simulink model "system_level_0317"  (R2025a)
settings: Solver=VariableStepAuto  StartTime=0.0  StopTime=600  RelTol=1e-3
libraries: simulink x6
settings Model: PacingRate=40  Creator=lynnyu  LastModifiedBy=lynnyu

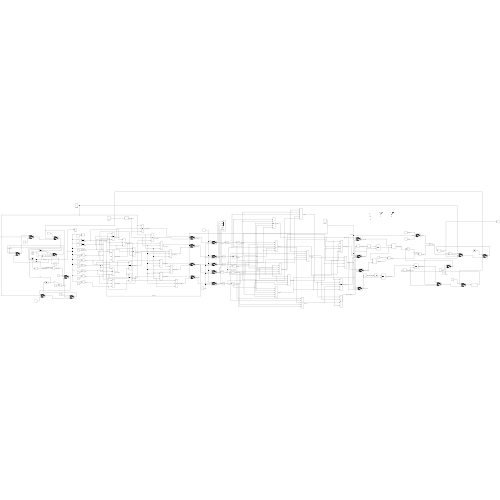
[thumbnail: Simulink's stored preview of the top-level diagram]
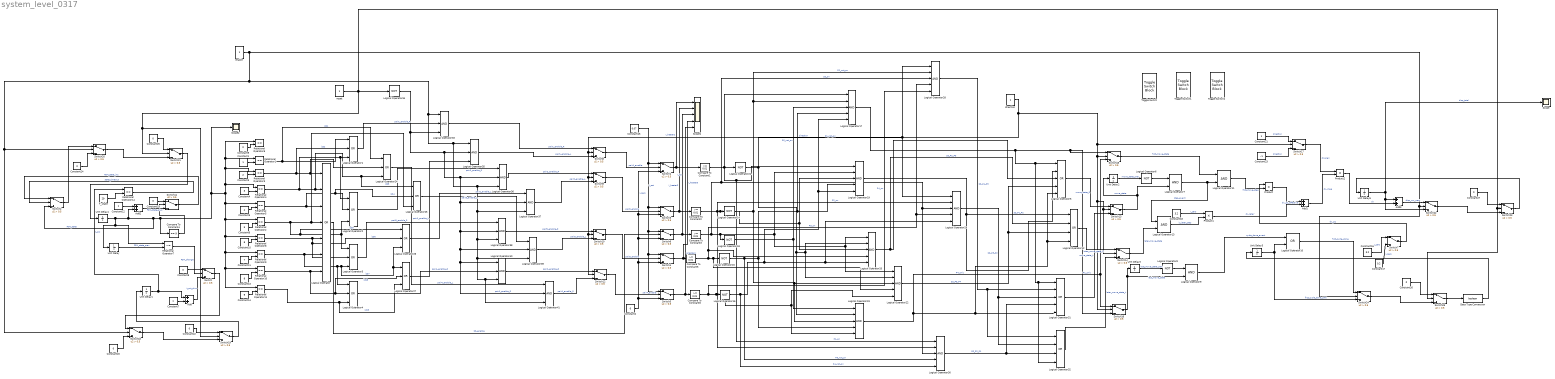
== system system_level_0317 ==
  Add{,1..3} (4 alike) : Sum
  Compare To Constant{1..3,5..6} (5 alike) : simulink/Logic and Bit Operations/Compare To Constant  relop=>=  const=0.01  OutDataTypeStr=boolean
  Compare To Constant4 : simulink/Logic and Bit Operations/Compare To Constant  relop===  const=9  OutDataTypeStr=boolean
  Constant{1,7,12,21} (4 alike) : Constant
  Constant10 : Constant  Value=6
  Constant11 : Constant  Value=7
  Constant13 : Constant  Value=8
  Constant14 : Constant  Value=9
  Constant15 : Constant  Value=0.07
  Constant16 : Constant  Value=3.2
  Constant17 : Constant  Value=0.2
  Constant18 : Constant  Value=3.2
  Constant{2,8..9,19..20,22,24..27} (10 alike) : Constant  Value=0
  Constant23 : Constant  Value=-1
  Constant3 : Constant  Value=2
  Constant4 : Constant  Value=3
  Constant5 : Constant  Value=4
  Constant6 : Constant  Value=5
  Data Type Conversion : DataTypeConversion  OutDataTypeStr=boolean  SaturateOnIntegerOverflow=off  RndMeth=Floor
  Logical Operator : Logic  Operator=OR  Inputs=7  AllPortsSameDT=off  OutDataTypeStr=boolean
  Logical Operator{1..4,24..27} (8 alike) : Logic  Operator=OR  Inputs=3  AllPortsSameDT=off  OutDataTypeStr=boolean
  Logical Operator10 : Logic  Operator=OR  AllPortsSameDT=off  OutDataTypeStr=boolean
  Logical Operator{7,9,11,13} (4 alike) : Logic  AllPortsSameDT=off  OutDataTypeStr=boolean
  Logical Operator12 : Logic  Operator=OR  Inputs=4  AllPortsSameDT=off  OutDataTypeStr=boolean
  Logical Operator{14..16,18,21,34} (6 alike) : Logic  Operator=NOT  Inputs=3  AllPortsSameDT=off  OutDataTypeStr=boolean
  Logical Operator{17,19..20,22..23,28..30} (8 alike) : Logic  Inputs=5  AllPortsSameDT=off  OutDataTypeStr=boolean
  Logical Operator31 : Logic  Operator=OR  Inputs=5  AllPortsSameDT=off  OutDataTypeStr=boolean
  Logical Operator32 : Logic  Operator=OR  Inputs=4  AllPortsSameDT=off  OutDataTypeStr=boolean
  Logical Operator{33,35..41} (8 alike) : Logic  Inputs=3  AllPortsSameDT=off  OutDataTypeStr=boolean
  Logical Operator5 : Logic  Operator=OR  Inputs=5  AllPortsSameDT=off  OutDataTypeStr=boolean
  Logical Operator6 : Logic  Operator=NOT  Inputs=5  AllPortsSameDT=off  OutDataTypeStr=boolean
  Logical Operator8 : Logic  Operator=NOT  Inputs=5  AllPortsSameDT=off  OutDataTypeStr=boolean
  Product : Product
  Product1 : Product
  Product2 : Product
  Relational Operator{1..6,8..11,14} (11 alike) : RelationalOperator  Operator===  OutDataTypeStr=boolean  RndMeth=Simplest  InputSameDT=off
  Relational Operator7 : RelationalOperator  Operator=~=  OutDataTypeStr=boolean  RndMeth=Simplest  InputSameDT=off
  Scope : Scope
      settings: ActiveDisplayYMinimum=-1  ActiveDisplayYMaximum=1
  Scope1 : Scope  NumInputPorts=5
      settings: ActiveDisplayYMinimum=-1  ActiveDisplayYMaximum=1
  Scope2 : Scope
      settings: ActiveDisplayYMinimum=-1.1249999999999998  ActiveDisplayYMaximum=10.125  DataLoggingVariableName=ScopeData2
  Switch{,1..25} (26 alike) : Switch  Criteria=u2 > Threshold  Threshold=0.5  SaturateOnIntegerOverflow=off  InputSameDT=off
  T_state : Constant  Value=29
  Toggle Switch : ToggleSwitchBlock
  Toggle Switch1 : ToggleSwitchBlock
  Toggle Switch2 : ToggleSwitchBlock
  Unit Delay : UnitDelay  SampleTime=-1  HasFrameUpgradeWarning=on
  Unit Delay{1..6} (6 alike) : UnitDelay  HasFrameUpgradeWarning=on
  direction : Constant
  enable : Constant
  reset : Constant
  wires:
  Constant1/1 -> Relational Operator1/2
  Constant3/1 -> Relational Operator3/2
  Constant4/1 -> Relational Operator4/2
  Constant5/1 -> Relational Operator5/2
  Unit Delay1/1 -> Add/1, Relational Operator14/1  "t_cnt"
  Constant7/1 -> Add/2
  Add/1 -> Switch/3  "t_cnt_plus"
  Constant8/1 -> Switch/1
  Relational Operator7/1 -> Switch/2  "FSM_change"
  Unit Delay/1 -> Relational Operator7/2  "FSM_state_prev"
  Relational Operator14/1 -> Switch2/2  "state_timeout"
  Add2/1 -> Switch11/3  "FSM_state_plus"
  Switch11/1 -> Switch2/1  "FSM_state_inc"
  T_state/1 -> Relational Operator14/2
  Compare To Constant4/1 -> Switch11/2
  Constant12/1 -> Add2/1
  Constant6/1 -> Relational Operator2/2
  Constant9/1 -> Relational Operator6/2
  Constant10/1 -> Relational Operator8/2
  Constant11/1 -> Relational Operator9/2
  Constant13/1 -> Relational Operator10/2
  Unit Delay4/1 -> Compare To Constant4/1, Scope2/1, Relational Operator4/1, Relational Operator3/1, Relational Operator1/1, Relational Operator6/1, Relational Operator11/1, Relational Operator10/1, Relational Operator9/1, Relational Operator8/1, Relational Operator2/1, Relational Operator5/1, Switch2/3, Add2/2, Unit Delay/1, Relational Operator7/1  "FSM_state"
  Constant14/1 -> Relational Operator11/2
  Relational Operator2/1 -> Logical Operator26/1, Logical Operator3/1, Logical Operator2/3, Logical Operator25/3, Logical Operator/4  "isS5"
  Relational Operator8/1 -> Logical Operator3/2, Logical Operator26/2, Logical Operator/5  "isS6"
  Relational Operator9/1 -> Logical Operator4/1, Logical Operator27/1, Logical Operator26/3, Logical Operator3/3, Logical Operator/6  "isS7"
  Relational Operator10/1 -> Logical Operator27/2, Logical Operator4/2, Logical Operator/7  "isS8"
  Relational Operator11/1 -> Logical Operator27/3, Logical Operator4/3  "isS9"
  Relational Operator1/1 -> Logical Operator24/1, Logical Operator1/1  "isS1"
  Relational Operator3/1 -> Logical Operator1/2, Logical Operator24/2, Logical Operator/1  "isS2"
  Relational Operator4/1 -> Logical Operator2/1, Logical Operator1/3, Logical Operator25/1, Logical Operator24/3, Logical Operator/2  "isS3"
  Relational Operator5/1 -> Logical Operator25/2, Logical Operator2/2, Logical Operator/3  "isS4"
  Logical Operator/1 -> Switch6/2  "SS_enable"
  Constant15/1 -> Switch1/1, Switch3/1, Switch6/1, Switch5/1, Switch4/1  "I_act"
  Constant2/1 -> Switch5/3, Switch4/3, Switch6/3, Switch3/3, Switch1/3  "I_zero"
  Switch1/1 -> Scope1/1, Compare To Constant1/1  "I_heater1"
  Switch3/1 -> Scope1/2, Compare To Constant2/1  "I_heater2"
  Switch4/1 -> Scope1/4, Compare To Constant5/1  "I_heater3"
  Switch5/1 -> Scope1/5, Compare To Constant6/1  "I_heater4"
  Switch6/1 -> Scope1/3, Compare To Constant3/1  "I_SS"
  Logical Operator5/1 -> Switch13/1  "move_state_R"
  Unit Delay2/1 -> Logical Operator6/1  "move_state_prev"
  Logical Operator6/1 -> Logical Operator7/1
  Unit Delay3/1 -> Logical Operator8/1  "last_move_state_prev"
  Logical Operator8/1 -> Logical Operator9/1
  Unit Delay5/1 -> Switch24/3, Logical Operator10/2  "first_cycle_done_prev"
  Logical Operator10/1 -> Switch24/1  "first_cycle_done"
  Logical Operator13/1 -> Product1/2  "is_later_step"
  Constant16/1 -> Switch7/1  "I_zero"
  Constant17/1 -> Switch7/3  "I_zero"
  Switch7/1 -> Product/1  "dx_S1"
  Product/1 -> Add1/1  "dx_S1_effective"
  Constant18/1 -> Product1/1  "I_zero"
  Unit Delay6/1 -> Switch22/3, Add3/1, Scope/1  "disp_total"
  Compare To Constant1/1 -> Logical Operator30/1, Logical Operator19/1, Logical Operator21/1, Logical Operator17/1  "P1_on"
  Compare To Constant2/1 -> Logical Operator30/2, Logical Operator29/2, Logical Operator14/1, Logical Operator20/3, Logical Operator19/3  "P2_on"
  Compare To Constant3/1 -> Logical Operator30/3, Logical Operator29/3, Logical Operator28/3, Logical Operator22/1, Logical Operator20/1, Logical Operator19/2, Logical Operator18/1  "SS_on"
  Compare To Constant5/1 -> Logical Operator29/4, Logical Operator28/4, Logical Operator20/4, Logical Operator15/1, Logical Operator22/4  "P3_on"
  Compare To Constant6/1 -> Logical Operator28/5, Logical Operator16/1, Logical Operator23/5, Logical Operator22/5  "P4_on"
  Logical Operator14/1 -> Logical Operator28/2, Logical Operator17/2, Logical Operator22/3, Logical Operator23/3  "P2_not_on"
  Logical Operator15/1 -> Logical Operator30/4, Logical Operator23/4, Logical Operator19/4, Logical Operator17/4  "P3_not_on"
  Logical Operator16/1 -> Logical Operator30/5, Logical Operator29/5, Logical Operator20/5, Logical Operator19/5, Logical Operator17/5  "P4_not_on"
  Logical Operator18/1 -> Logical Operator17/3, Logical Operator23/1  "SS_not_on"
  Logical Operator19/1 -> Logical Operator5/2, Logical Operator12/1  "SS_P1_P2"
  Logical Operator21/1 -> Logical Operator23/2, Logical Operator22/2, Logical Operator20/2, Logical Operator28/1, Logical Operator29/1  "P1_not_on"
  Logical Operator20/1 -> Logical Operator5/3, Logical Operator12/2  "SS_P2_P3"
  Logical Operator22/1 -> Logical Operator12/3, Logical Operator5/4  "SS_P3_P4"
  Logical Operator23/1 -> Switch16/1, Switch15/3, Logical Operator12/4, Logical Operator5/5, Logical Operator31/5  "P4_only"
  Logical Operator17/1 -> Switch15/1, Switch16/3, Logical Operator32/4, Logical Operator31/1, Logical Operator5/1  "P1_only"
  Logical Operator7/1 -> Logical Operator13/1, Logical Operator11/2  "step_event"
  Logical Operator11/1 -> Product/2  "first_move_step"
  Logical Operator9/1 -> Logical Operator10/1  "cycle_done_event"
  Product1/1 -> Add1/2  "dx_later'"
  Constant19/1 -> Switch11/1
  Switch8/1 -> Switch1/2  "pair1_enable"
  Switch9/1 -> Switch3/2  "pair2_enable"
  Switch10/1 -> Switch4/2  "pair3_enable"
  Switch12/1 -> Switch5/2  "pair4_enable"
  Logical Operator28/1 -> Logical Operator32/1, Logical Operator31/2  "SS_P4_P3"
  Logical Operator29/1 -> Logical Operator32/2, Logical Operator31/3  "SS_P3_P2"
  Logical Operator30/1 -> Logical Operator31/4, Logical Operator32/3  "SS_P2_P1"
  Logical Operator31/1 -> Switch13/3  "move_state_L"
  Logical Operator32/1 -> Switch14/3  "later_move_state_L"
  Switch13/1 -> Unit Delay2/1, Logical Operator7/2  "move_state"
  Switch14/1 -> Logical Operator13/2  "later_move_state"
  Logical Operator12/1 -> Switch14/1  "later_move_state_R"
  Switch15/1 -> Logical Operator11/1  "first_move_state"
  Switch16/1 -> Logical Operator9/2, Unit Delay3/1  "last_move_state"
  Constant21/1 -> Switch17/1  "direction"
  direction/1 -> Switch12/2, Switch10/2, Switch9/2, Switch8/2, Switch17/2, Switch14/2, Switch13/2, Switch16/2, Switch15/2  "direction"
  Constant23/1 -> Switch17/3  "direction"
  Switch17/1 -> Product2/1  "dir_sign"
  Add1/1 -> Product2/2  "dx_mag"
  Product2/1 -> Add3/2  "dx"
  Switch19/1 -> Unit Delay1/1
  Switch/1 -> Switch18/1
  Constant20/1 -> Switch18/3
  reset/1 -> Switch25/2, Switch23/2, Logical Operator34/1, Switch21/2, Switch19/2
  Constant24/1 -> Switch20/3
  Switch2/1 -> Switch20/1
  Switch21/1 -> Unit Delay4/1
  Logical Operator1/1 -> Logical Operator33/2  "pair1_enable_R"
  Logical Operator33/1 -> Switch8/1  "pair1_enable_R"
  Logical Operator34/1 -> Logical Operator41/2, Logical Operator40/1, Logical Operator39/2, Logical Operator38/2, Logical Operator37/2, Logical Operator36/2, Logical Operator35/2, Logical Operator33/3  "pair1_enable_R"
  Logical Operator27/1 -> Logical Operator35/3  "pair1_enable_L"
  Logical Operator35/1 -> Switch8/3  "pair1_enable_L"
  Logical Operator2/1 -> Logical Operator36/1  "pair2_enable_R"
  Logical Operator36/1 -> Switch9/1  "pair2_enable_R"
  Logical Operator26/1 -> Logical Operator37/1  "pair2_enable_L"
  Logical Operator37/1 -> Switch9/3  "pair2_enable_L"
  Logical Operator38/1 -> Switch10/1  "pair3_enable_R"
  Logical Operator3/1 -> Logical Operator38/1  "pair3_enable_R"
  Logical Operator25/1 -> Logical Operator39/1  "pair3_enable_L"
  Logical Operator39/1 -> Switch10/3  "pair3_enable_L"
  Logical Operator40/1 -> Switch12/1  "pair1_enable_R"
  Logical Operator4/1 -> Logical Operator40/2  "pair4_enable_R"
  Logical Operator24/1 -> Logical Operator41/1  "pair4_enable_L"
  Logical Operator41/1 -> Switch12/3  "pair1_enable_R"
  Add3/1 -> Switch22/1  "disp_run_next"
  enable/1 -> Switch24/2, Switch22/2, Switch18/2, Switch20/2, Logical Operator33/1, Logical Operator41/3, Logical Operator40/3, Logical Operator39/3, Logical Operator38/3, Logical Operator37/3, Logical Operator36/3, Logical Operator35/1
  Switch23/1 -> Unit Delay6/1
  Constant27/1 -> Switch23/1
  Switch22/1 -> Switch23/3
  Constant26/1 -> Switch25/1
  Switch24/1 -> Switch25/3
  Switch25/1 -> Data Type Conversion/1
  Data Type Conversion/1 -> Unit Delay5/1
  Constant22/1 -> Switch19/1
  Switch18/1 -> Switch19/3
  Constant25/1 -> Switch21/1
  Switch20/1 -> Switch21/3
